simulink library "dspSarDemoLib"  (Simulink 8.3)
settings: Solver=ode45  SolverMode=SingleTasking  StartTime=0.0  StopTime=10.0  RelTol=1e-3
libraries: dspxfrm3 x2
settings Model: FPTRunName=Active  Creator=The MathWorks Inc.  ExtModeAutoUpdateStatusClock=off

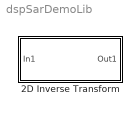
== system dspSarDemoLib ==
  2D Inverse Transform : Subsystem  mask(2D Inverse Transform){}
      mask help: Performs a 2-D Inverse FFT of the input.
      mask Display: disp('2-D Inverse\nTransform');

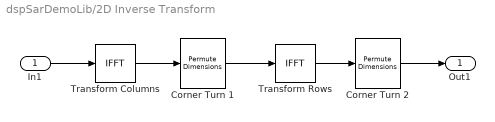
== system dspSarDemoLib/2D Inverse Transform ==
  In1 : Inport
  Corner Turn 1 : PermuteDimensions
  Corner Turn 2 : PermuteDimensions
  Transform Columns : dspxfrm3/IFFT  CompMethod=Table lookup  TableOpt=NEW  TableOptActive=Speed  BitRevOrder=off  cs_in=off  SkipNorm=on  InheritFFTLength=on  FFTLength=64  WrapInput=on  mode=Complex  outSamplingMode=Sample based  RowConvenienceOn=on  FFTImplementation=Auto  firstCoeffDataTypeStr=Inherit: Same word length as input  firstCoeffLastDataTypeStr=Inherit: Same word length as input  outputMin=[]  outputMax=[]  roundingMode=Floor  overflowMode=off
  Transform Rows : dspxfrm3/IFFT  CompMethod=Table lookup  TableOpt=NEW  TableOptActive=Speed  BitRevOrder=off  cs_in=off  SkipNorm=on  InheritFFTLength=on  FFTLength=64  WrapInput=on  mode=Complex  outSamplingMode=Sample based  RowConvenienceOn=on  FFTImplementation=Auto  firstCoeffDataTypeStr=Inherit: Same word length as input  firstCoeffLastDataTypeStr=Inherit: Same word length as input  outputMin=[]  outputMax=[]  roundingMode=Floor  overflowMode=off
  Out1 : Outport
  wires:
  In1/1 -> Transform Columns/1
  Transform Columns/1 -> Corner Turn 1/1
  Transform Rows/1 -> Corner Turn 2/1
  Corner Turn 1/1 -> Transform Rows/1
  Corner Turn 2/1 -> Out1/1
